simulink model "Flexible_Beam_Compare"  (R2016a)
settings: Solver=ode23t  StartTime=0.0  StopTime=10  MaxStep=5e-3  RelTol=1e-3  AbsTol=1e-3
PreLoadFcn:
  | Rigid_BoB = Simulink.Variant('Rigid_Body == 1');
  | Rigid_Link = Simulink.Variant('Rigid_Body == 2');
  | Rigid_Body = 1;
PostLoadFcn:
  | warning off Simulink:Engine:UsingDefaultMaxStepSize
  | warning off sm:compiler:topologyAnalysis:OnePortForceBlockGrounded
  | warning off Simulink:Parameters:ASTReadOnlyIfCompiledMaskField
  | warning off Simulink:Engine:SaveWithParameterizedLinks_Warning
  | warning off Simulink:Engine:OutputNotConnected
  | warning off Simulink:Engine:InputNotConnected
InitFcn:
  | %if ~exist('linsys_beam_fixfree','var') ||~exist('linsys_beam_rotfree','var')
  |    load SS_Damping_1e7.mat
  |    disp('State Space Models does not exist in workspace, loading presaved SS models')
  | %end
undefined symbols (not defined in the file or in its folder): beam_length, beam_wall, beam_width, density, element_length, Extr_Data_Box, gravity, Heavy_Weight, num_elem, X, Y, Z
undefined symbols (not defined in the file): Damping, kbendingx, kbendingy, kelongz, ktwistz, shearM, youngsM
libraries: sm_lib x240, nesl_utility x9, cstblocks x1
(part 1 of 7)
Description:
  | Copyright 2014-2016 The MathWorks, Inc.
settings Model: TunableVars=Heavy_Weight  TunableVarsStorageClass=Auto  Creator=smiller  LastModifiedBy=smiller
settings SolverCC: ZeroCrossAlgorithm=Adaptive
settings DataIOCC: LimitDataPoints=on  SaveFormat=Array
settings OptimizationCC: DefaultParameterBehavior=Inlined
settings DebuggingCC: AlgebraicLoopMsg=error  UnderspecifiedInitializationDetection=Classic  MergeDetectMultiDrivingBlocksExec=none  SolverPrmCheckMsg=warning  AllowSymbolicDim=off  StateNameClashWarn=warning
settings HardwareCC: ProdBitPerPointer=32  ProdLargestAtomicFloat=None  ProdIntDivRoundTo=Undefined  ProdEndianess=Unspecified  ProdWordSize=32  ProdHWDeviceType=32-bit Generic  TargetBitPerPointer=64  TargetLongLongMode=on  TargetIntDivRoundTo=Zero  TargetEndianess=LittleEndian  TargetWordSize=64  TargetHWDeviceType=MATLAB Host  ProdEqTarget=off
settings ModelReferenceCC: PropagateSignalLabelsOutOfModel=off
settings RTWCC: SystemTargetFile=rsim.tlc  TemplateMakefile=rsim_default_tmf  Description=Rapid Simulation Target
settings RSimTargetCC: ERTMultiwordTypeDef=System defined  ERTMultiwordLength=256
settings ConfigComp: CovModelRefEnable=Off  CovSFcnEnable=off
settings SimscapeCC: SimscapeLogLimitData=off
settings ConfigurationSet: Description=SimMechanics 2G
settings DiagnosticsConfigSet: SimMechanicsUnconnectedFramePorts=none  SimMechanicsRigidlyBoundBlock=warning
settings ExplorerConfigSet: InternalSimMechanicsExplorerSettings="<ExplorerConfiguration><canonicalview>default</canonicalview><AnimationSetting><BasePlaybackSpeed>1.0</BasePlaybackSpeed><PlaybackSpeedFactor>1.0</PlaybackSpeedFactor></AnimationSetting><TilePanel><TileInfo><Tiles Columns=\"1\" Count=\"1\" Rows=\"1\"><Column Left=\"2\" Weight=\"1\"/><Column Left=\"626\"/><Row Top=\"2\" Weight=\"1\"/><Row Top=\"393\"/><Tile Height=\"1\" Width=\"1\" X=\"0\" Y=\"0\"/></Tiles></TileInfo><SceneInfo><SceneViewer><BGColor><R>0.60000002384185791</R><G>0.60000002384185791</G><B>0.60000002384185791</B></BGColor><Camera><Position><X>49.330755486805451</X><Y>-0.55803913686158779</Y><Z>2.4998328760631781</Z></Position><Center><X>15.534556771714037</X><Y>-0.93059923918877141</Y><Z>0.031810436074220405</Z></Center><Up><X>-0.011334240993120652</X><Y>0.99992667770693056</Y><Z>0.004263119877513607</Z></Up><Left>-2.2154408151596012</Left><Right>2.2154408151596012</Right><Bottom>-1.878380911550241</Bottom><Top>1.878380911550241</Top></Camera></SceneViewer></SceneInfo></TilePanel></ExplorerConfiguration>"

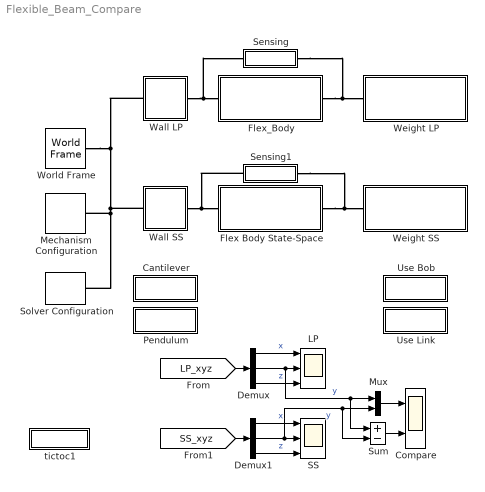
== system Flexible_Beam_Compare ==
  Cantilever : Subsystem
      settings: OpenFcn=|
      | set_param([bdroot '/Wall LP'],'OverrideUsingVariant','Fixed');
      | set_param([bdroot '/Wall SS'],'OverrideUsingVariant','Fixed');
      | 
      | LTIpth = find_system(bdroot,'ReferenceBlock','cstblocks/LTI System');
      | set_param(char(LTIpth),'sys','linsys_beam_fixfree');
      mask Display: disp('Cantilever');
  Compare : Scope  NumInputPorts=2
  Demux : Demux  Outputs=3
  Demux1 : Demux  Outputs=3
  Flex Body State-Space : Subsystem
      mask Display:
      | image(imread('SS_Beam.png'));
      | color red
      | port_label('LConn',1,'B');
      | port_label('RConn',1,'F');
  Flex_Body : Subsystem  mask(Flexible Body){rho=density, youngsM=youngsM, shearM=shearM, numelem=num_elem, beam_length=beam_length, beam_width=beam_width, beam_wall=beam_wall, b=Damping}
      mask prompts: rho "Material Density (kg/(m^3)"; youngsM "Modulus of Elasticity (N/m2)"; shearM "Shear Modulus (N/m2)"; numelem "Number of elements"; beam_length "Beam Length (m)"; beam_width "Beam Width & Height (m)"; beam_wall "Beam Wall Thickness(m)"; b "Damping Constant (Nm/rad.s)"
      mask help:
      | Models a flexible hollow square beam based on lumped parameter method.
      | Number of flexible elements, material properties as well as beam
      | dimension can be varied from mask parameters.
      mask init:
      | [kbendingx, kbendingy, ktwistz, kelongz, length] = Compute_GFE_Prop(rho, youngsM, shearM, numelem, beam_length, beam_width,beam_wall);
      | thisblock = gcb;
      | anno = ['No of Elem: ' num2str(numelem)];
      | set_param(thisblock, 'AttributesFormatString',anno);
      | if numelem <1
      |     error('Number of Flexible elements should be greater than 0')
      | end
      | prev_flex_bod = find_system(gcb,'LookUnderMasks','all','RegExp','on','Name','Flex_Elem_*');
      | if ~isempty(prev_flex_bod)
      |     delete_block(prev_flex_bod(1:end))
      | end
      | linehan = find_system(thisblock,'LookUnderMasks','all','FindAll','on','type','line');
      | if ~isempty(linehan)
      |     delete_line(linehan)
      | end
      | blk_or = [100 155 140 195];
      | set_param([thisblock '/B'],'Position',blk_or)
      | set_param([thisblock '/' sprintf('Transform\nBeamX')],'Position',blk_or+[80 0 80 0])
      | add_line(thisblock,['B/Rconn1'],[sprintf('Transform\nBeamX') '/Lconn1'],'autorouting','on');
      | add_block('FlexBeamElement_MS2G_Lib/Bend_Simple',[thisblock '/Flex_Elem_' num2str(1)],'Position',blk_or+[80 0 80 0]*2)
      | add_line(thisblock,[sprintf('Transform\nBeamX') '/Rconn1'],['Flex_Elem_' num2str(1) '/Lconn1'],'autorouting','on');
      | set_param([thisblock '/Flex_Elem_' num2str(1)], 'LinkStatus', 'none')
      | state_order{1} = [thisblock '/Flex_Elem_' num2str(1) '/Revolute Joint'];
      | for i = 2:1:numelem
      |     add_block('FlexBeamElement_MS2G_Lib/Bend_Simple',[thisblock '/Flex_Elem_' num2str(i)],'Position',blk_or+(i+1)*[80 0 80 0])
      |     add_line(thisblock,['Flex_Elem_' num2str(i-1) '/Rconn1'],['Flex_Elem_' num2str(i) '/Lconn1'],'autorouting','on');
      |     set_param([thisblock '/Flex_Elem_' num2str(i)], 'LinkStatus', 'none')
      |     state_order{i} = [thisblock '/Flex_Elem_' num2str(i) '/Revolute Joint'];
      | end
      | set_param([thisblock '/F'],'Position',blk_or+ (numelem+2)*[80 0 80 0]);
      | add_line(thisblock,['Flex_Elem_' num2str(numelem) '/Rconn1'],['F/Rconn1'],'autorouting','on');
      | assignin('base','State_order',state_order)
      settings: AttributesFormatString=No of Elem: 30  CopyFcn=set_param(gcb, 'LinkStatus', 'none')
      mask Display:
      | image(imread('Flexible_Beam.png'));
      | color red
      | port_label('LConn',1,'B');
      | port_label('RConn',1,'F');
  LP : Scope  NumInputPorts=3
  Mechanism Configuration : sm_lib/Utilities/Mechanism Configuration  UniformGravity=Constant  GravityVector=gravity  GravityUnits=m/s^2  LinearizationDelta=0.001
  Mux : Mux  Inputs=2
  Pendulum : Subsystem
      settings: OpenFcn=|
      | set_param([bdroot '/Wall LP'],'OverrideUsingVariant','Rotate');
      | set_param([bdroot '/Wall SS'],'OverrideUsingVariant','Rotate');
      | 
      | LTIpth = find_system(bdroot,'ReferenceBlock','cstblocks/LTI System');
      | set_param(char(LTIpth),'sys','linsys_beam_rotfree');
      mask Display: disp('Pendulum');
  SS : Scope  NumInputPorts=3
  Sensing : Subsystem
      mask Display: disp('S')
  Sensing1 : Subsystem
      mask Display: disp('S')
  Solver Configuration : nesl_utility/Solver Configuration  PhysicalDomain=network_engine_domain  SubClassName=solver  LeftPortType=input  RightPortType=generic  Accelerate=off  Tones=[]  Harmonics=[]  SimulateNoise=off  Profile=off  UseLocalSampling=off  EnableSwitchedLinearOptims=on  FrequencyDomain=off  UseCCode=off  RelTol=0.001  AbsTol=1e-06  MinStep=1e-09  ToWorkspace=off  RevertToSquareIcSolve=off  NumHomotopyIterations=100  PhasorMode=off  PhasorModeNumHarmonics=1  OverrideAbsTol=off  DoDC=off  ResidualTolerance=1e-09  UseLocalSolver=off  LocalSolverChoice=NE_BACKWARD_EULER_ADVANCER  LocalSolverSampleTime=0.001  DoFixedCost=off  MaxNonlinIter=3  MaxModeIter=2  LinearAlgebra=Sparse  DelaysMemoryBudget=1024  AutomaticFiltering=on  FilteringTimeConstant=0.001
  Sum : Sum  Inputs=+-
  Use Bob : Subsystem
      settings: OpenFcn=|
      | set_param([bdroot '/Weight LP'],'OverrideUsingVariant','Bob');
      | set_param([bdroot '/Weight SS'],'OverrideUsingVariant','Bob');
      mask Display: disp('Use Bob');
  Use Link : Subsystem
      settings: OpenFcn=|
      | set_param([bdroot '/Weight LP'],'OverrideUsingVariant','Link');
      | set_param([bdroot '/Weight SS'],'OverrideUsingVariant','Link');
      mask Display: disp('Use Link');
  Wall LP : Subsystem  Variant=on  OverrideUsingVariant=Fixed
      mask Display:
      | if strcmp(get_param(gcb,'ActiveVariant'),'Fixed')
      |     image(imread('Weld_Image.png'))
      | else
      |     image(imread('Rev_Image.png'))
      | end
      | color red
      | port_label('LConn',1,'B');
      | port_label('Rconn',1,'F');
  Wall SS : Subsystem  Variant=on  OverrideUsingVariant=Fixed
      mask Display:
      | if strcmp(get_param(gcb,'ActiveVariant'),'Fixed')
      |     image(imread('Weld_Image.png'))
      | else
      |     image(imread('Rev_Image.png'))
      | end
      | color red
      | port_label('LConn',1,'B');
      | port_label('Rconn',1,'F');
  Weight LP : Subsystem  Variant=on  OverrideUsingVariant=Bob
      mask Display:
      | if strcmp(get_param(gcb,'ActiveVariant'),'Bob')
      |     image(imread('BOB_LP.png'))
      | else
      |     image(imread('Link.png'))
      | end
      | color red
      | port_label('LConn',1,'B');
      | port_label('Rconn',1,'F');
  Weight SS : Subsystem  Variant=on  OverrideUsingVariant=Bob
      mask Display:
      | if strcmp(get_param(gcb,'ActiveVariant'),'Bob')
      |     image(imread('BOB.png'))
      | else
      |     image(imread('Link.png'))
      | end
      | color red
      | port_label('LConn',1,'B');
      | port_label('Rconn',1,'F');
  World Frame : sm_lib/Frames and Transforms/World Frame
  tictoc1 : Subsystem
      settings: OpenFcn=open('Flexible_Beam_Demo_Script.html')
      mask Display: disp('Script')
  wires:
  Demux/1 -> LP/1  "x"
  Demux/2 -> Sum/1, Mux/1, LP/2  "y"
  Demux/3 -> LP/3  "z"
  Demux1/1 -> SS/1  "x"
  Demux1/2 -> SS/2, Sum/2, Mux/2  "y"
  Demux1/3 -> SS/3  "z"
  Mux/1 -> Compare/1
  Sum/1 -> Compare/2
  [LP_xyz] -> Demux/1
  [SS_xyz] -> Demux1/1
  connections:
  Solver Configuration/RConn1 -- Wall LP/LConn1 -- World Frame/RConn1 -- Wall SS/LConn1 -- Mechanism Configuration/RConn1
  Sensing/LConn1 -- Flex_Body/RConn1 -- Weight LP/LConn1
  Flex Body State-Space/RConn1 -- Sensing1/LConn1 -- Weight SS/LConn1
  Wall LP/RConn1 -- Flex_Body/LConn1 -- Sensing/RConn1
  Wall SS/RConn1 -- Sensing1/RConn1 -- Flex Body State-Space/LConn1

== system Flexible_Beam_Compare/Cantilever ==

== system Flexible_Beam_Compare/Flex Body State-Space ==
  Deflection Joint : Subsystem
  Rigid Body : Subsystem
  State-Space Model : Subsystem
  B : PMIOPort  Port=1  Side=Left
  F : PMIOPort  Port=2  Side=Right
  connections:
  Deflection Joint/RConn2 -- F/RConn1
  Rigid Body/LConn1 -- B/RConn1
  Deflection Joint/LConn2 -- Rigid Body/RConn1
  State-Space Model/RConn1 -- Deflection Joint/LConn1
  State-Space Model/LConn1 -- Deflection Joint/RConn1

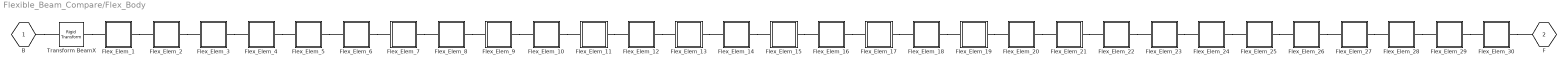
== system Flexible_Beam_Compare/Flex_Body ==
  Flex_Elem_1 : Subsystem  mask{length=length, rho=rho, beam_width=beam_width, beam_wall=beam_wall, kbendingx=kbendingx, kbendingy=kbendingy, kbendingz=ktwistz, kelongz=kelongz, b=b}
      mask prompts: length "Beam Length (m)"; rho "Material Density (kg/(m^3)"; beam_width "Beam Width & Height (m)"; beam_wall "Beam Wall Thickness (m)"; kbendingx "Bending Spring Constant about X(Nm/rad)"; kbendingy "Bending Spring Constant about Y(Nm/rad)"; kbendingz "Twist Spring Constant about Z(Nm/rad)"; kelongz "Elongation Spring Constant about Z(N/m)"; b "Damping Constant (Nm/rad.s)"
  Flex_Elem_10 : Subsystem  mask{length=length, rho=rho, beam_width=beam_width, beam_wall=beam_wall, kbendingx=kbendingx, kbendingy=kbendingy, kbendingz=ktwistz, kelongz=kelongz, b=b}
      mask prompts: length "Beam Length (m)"; rho "Material Density (kg/(m^3)"; beam_width "Beam Width & Height (m)"; beam_wall "Beam Wall Thickness (m)"; kbendingx "Bending Spring Constant about X(Nm/rad)"; kbendingy "Bending Spring Constant about Y(Nm/rad)"; kbendingz "Twist Spring Constant about Z(Nm/rad)"; kelongz "Elongation Spring Constant about Z(N/m)"; b "Damping Constant (Nm/rad.s)"
  Flex_Elem_11 : Subsystem  mask{length=length, rho=rho, beam_width=beam_width, beam_wall=beam_wall, kbendingx=kbendingx, kbendingy=kbendingy, kbendingz=ktwistz, kelongz=kelongz, b=b}
      mask prompts: length "Beam Length (m)"; rho "Material Density (kg/(m^3)"; beam_width "Beam Width & Height (m)"; beam_wall "Beam Wall Thickness (m)"; kbendingx "Bending Spring Constant about X(Nm/rad)"; kbendingy "Bending Spring Constant about Y(Nm/rad)"; kbendingz "Twist Spring Constant about Z(Nm/rad)"; kelongz "Elongation Spring Constant about Z(N/m)"; b "Damping Constant (Nm/rad.s)"
  Flex_Elem_12 : Subsystem  mask{length=length, rho=rho, beam_width=beam_width, beam_wall=beam_wall, kbendingx=kbendingx, kbendingy=kbendingy, kbendingz=ktwistz, kelongz=kelongz, b=b}
      mask prompts: length "Beam Length (m)"; rho "Material Density (kg/(m^3)"; beam_width "Beam Width & Height (m)"; beam_wall "Beam Wall Thickness (m)"; kbendingx "Bending Spring Constant about X(Nm/rad)"; kbendingy "Bending Spring Constant about Y(Nm/rad)"; kbendingz "Twist Spring Constant about Z(Nm/rad)"; kelongz "Elongation Spring Constant about Z(N/m)"; b "Damping Constant (Nm/rad.s)"
  Flex_Elem_13 : Subsystem  mask{length=length, rho=rho, beam_width=beam_width, beam_wall=beam_wall, kbendingx=kbendingx, kbendingy=kbendingy, kbendingz=ktwistz, kelongz=kelongz, b=b}
      mask prompts: length "Beam Length (m)"; rho "Material Density (kg/(m^3)"; beam_width "Beam Width & Height (m)"; beam_wall "Beam Wall Thickness (m)"; kbendingx "Bending Spring Constant about X(Nm/rad)"; kbendingy "Bending Spring Constant about Y(Nm/rad)"; kbendingz "Twist Spring Constant about Z(Nm/rad)"; kelongz "Elongation Spring Constant about Z(N/m)"; b "Damping Constant (Nm/rad.s)"
  Flex_Elem_14 : Subsystem  mask{length=length, rho=rho, beam_width=beam_width, beam_wall=beam_wall, kbendingx=kbendingx, kbendingy=kbendingy, kbendingz=ktwistz, kelongz=kelongz, b=b}
      mask prompts: length "Beam Length (m)"; rho "Material Density (kg/(m^3)"; beam_width "Beam Width & Height (m)"; beam_wall "Beam Wall Thickness (m)"; kbendingx "Bending Spring Constant about X(Nm/rad)"; kbendingy "Bending Spring Constant about Y(Nm/rad)"; kbendingz "Twist Spring Constant about Z(Nm/rad)"; kelongz "Elongation Spring Constant about Z(N/m)"; b "Damping Constant (Nm/rad.s)"
  Flex_Elem_15 : Subsystem  mask{length=length, rho=rho, beam_width=beam_width, beam_wall=beam_wall, kbendingx=kbendingx, kbendingy=kbendingy, kbendingz=ktwistz, kelongz=kelongz, b=b}
      mask prompts: length "Beam Length (m)"; rho "Material Density (kg/(m^3)"; beam_width "Beam Width & Height (m)"; beam_wall "Beam Wall Thickness (m)"; kbendingx "Bending Spring Constant about X(Nm/rad)"; kbendingy "Bending Spring Constant about Y(Nm/rad)"; kbendingz "Twist Spring Constant about Z(Nm/rad)"; kelongz "Elongation Spring Constant about Z(N/m)"; b "Damping Constant (Nm/rad.s)"
  Flex_Elem_16 : Subsystem  mask{length=length, rho=rho, beam_width=beam_width, beam_wall=beam_wall, kbendingx=kbendingx, kbendingy=kbendingy, kbendingz=ktwistz, kelongz=kelongz, b=b}
      mask prompts: length "Beam Length (m)"; rho "Material Density (kg/(m^3)"; beam_width "Beam Width & Height (m)"; beam_wall "Beam Wall Thickness (m)"; kbendingx "Bending Spring Constant about X(Nm/rad)"; kbendingy "Bending Spring Constant about Y(Nm/rad)"; kbendingz "Twist Spring Constant about Z(Nm/rad)"; kelongz "Elongation Spring Constant about Z(N/m)"; b "Damping Constant (Nm/rad.s)"
  Flex_Elem_17 : Subsystem  mask{length=length, rho=rho, beam_width=beam_width, beam_wall=beam_wall, kbendingx=kbendingx, kbendingy=kbendingy, kbendingz=ktwistz, kelongz=kelongz, b=b}
      mask prompts: length "Beam Length (m)"; rho "Material Density (kg/(m^3)"; beam_width "Beam Width & Height (m)"; beam_wall "Beam Wall Thickness (m)"; kbendingx "Bending Spring Constant about X(Nm/rad)"; kbendingy "Bending Spring Constant about Y(Nm/rad)"; kbendingz "Twist Spring Constant about Z(Nm/rad)"; kelongz "Elongation Spring Constant about Z(N/m)"; b "Damping Constant (Nm/rad.s)"
  Flex_Elem_18 : Subsystem  mask{length=length, rho=rho, beam_width=beam_width, beam_wall=beam_wall, kbendingx=kbendingx, kbendingy=kbendingy, kbendingz=ktwistz, kelongz=kelongz, b=b}
      mask prompts: length "Beam Length (m)"; rho "Material Density (kg/(m^3)"; beam_width "Beam Width & Height (m)"; beam_wall "Beam Wall Thickness (m)"; kbendingx "Bending Spring Constant about X(Nm/rad)"; kbendingy "Bending Spring Constant about Y(Nm/rad)"; kbendingz "Twist Spring Constant about Z(Nm/rad)"; kelongz "Elongation Spring Constant about Z(N/m)"; b "Damping Constant (Nm/rad.s)"
  Flex_Elem_19 : Subsystem  mask{length=length, rho=rho, beam_width=beam_width, beam_wall=beam_wall, kbendingx=kbendingx, kbendingy=kbendingy, kbendingz=ktwistz, kelongz=kelongz, b=b}
      mask prompts: length "Beam Length (m)"; rho "Material Density (kg/(m^3)"; beam_width "Beam Width & Height (m)"; beam_wall "Beam Wall Thickness (m)"; kbendingx "Bending Spring Constant about X(Nm/rad)"; kbendingy "Bending Spring Constant about Y(Nm/rad)"; kbendingz "Twist Spring Constant about Z(Nm/rad)"; kelongz "Elongation Spring Constant about Z(N/m)"; b "Damping Constant (Nm/rad.s)"
  Flex_Elem_2 : Subsystem  mask{length=length, rho=rho, beam_width=beam_width, beam_wall=beam_wall, kbendingx=kbendingx, kbendingy=kbendingy, kbendingz=ktwistz, kelongz=kelongz, b=b}
      mask prompts: length "Beam Length (m)"; rho "Material Density (kg/(m^3)"; beam_width "Beam Width & Height (m)"; beam_wall "Beam Wall Thickness (m)"; kbendingx "Bending Spring Constant about X(Nm/rad)"; kbendingy "Bending Spring Constant about Y(Nm/rad)"; kbendingz "Twist Spring Constant about Z(Nm/rad)"; kelongz "Elongation Spring Constant about Z(N/m)"; b "Damping Constant (Nm/rad.s)"
  Flex_Elem_20 : Subsystem  mask{length=length, rho=rho, beam_width=beam_width, beam_wall=beam_wall, kbendingx=kbendingx, kbendingy=kbendingy, kbendingz=ktwistz, kelongz=kelongz, b=b}
      mask prompts: length "Beam Length (m)"; rho "Material Density (kg/(m^3)"; beam_width "Beam Width & Height (m)"; beam_wall "Beam Wall Thickness (m)"; kbendingx "Bending Spring Constant about X(Nm/rad)"; kbendingy "Bending Spring Constant about Y(Nm/rad)"; kbendingz "Twist Spring Constant about Z(Nm/rad)"; kelongz "Elongation Spring Constant about Z(N/m)"; b "Damping Constant (Nm/rad.s)"
  Flex_Elem_21 : Subsystem  mask{length=length, rho=rho, beam_width=beam_width, beam_wall=beam_wall, kbendingx=kbendingx, kbendingy=kbendingy, kbendingz=ktwistz, kelongz=kelongz, b=b}
      mask prompts: length "Beam Length (m)"; rho "Material Density (kg/(m^3)"; beam_width "Beam Width & Height (m)"; beam_wall "Beam Wall Thickness (m)"; kbendingx "Bending Spring Constant about X(Nm/rad)"; kbendingy "Bending Spring Constant about Y(Nm/rad)"; kbendingz "Twist Spring Constant about Z(Nm/rad)"; kelongz "Elongation Spring Constant about Z(N/m)"; b "Damping Constant (Nm/rad.s)"
  Flex_Elem_22 : Subsystem  mask{length=length, rho=rho, beam_width=beam_width, beam_wall=beam_wall, kbendingx=kbendingx, kbendingy=kbendingy, kbendingz=ktwistz, kelongz=kelongz, b=b}
      mask prompts: length "Beam Length (m)"; rho "Material Density (kg/(m^3)"; beam_width "Beam Width & Height (m)"; beam_wall "Beam Wall Thickness (m)"; kbendingx "Bending Spring Constant about X(Nm/rad)"; kbendingy "Bending Spring Constant about Y(Nm/rad)"; kbendingz "Twist Spring Constant about Z(Nm/rad)"; kelongz "Elongation Spring Constant about Z(N/m)"; b "Damping Constant (Nm/rad.s)"
  Flex_Elem_23 : Subsystem  mask{length=length, rho=rho, beam_width=beam_width, beam_wall=beam_wall, kbendingx=kbendingx, kbendingy=kbendingy, kbendingz=ktwistz, kelongz=kelongz, b=b}
      mask prompts: length "Beam Length (m)"; rho "Material Density (kg/(m^3)"; beam_width "Beam Width & Height (m)"; beam_wall "Beam Wall Thickness (m)"; kbendingx "Bending Spring Constant about X(Nm/rad)"; kbendingy "Bending Spring Constant about Y(Nm/rad)"; kbendingz "Twist Spring Constant about Z(Nm/rad)"; kelongz "Elongation Spring Constant about Z(N/m)"; b "Damping Constant (Nm/rad.s)"
  Flex_Elem_24 : Subsystem  mask{length=length, rho=rho, beam_width=beam_width, beam_wall=beam_wall, kbendingx=kbendingx, kbendingy=kbendingy, kbendingz=ktwistz, kelongz=kelongz, b=b}
      mask prompts: length "Beam Length (m)"; rho "Material Density (kg/(m^3)"; beam_width "Beam Width & Height (m)"; beam_wall "Beam Wall Thickness (m)"; kbendingx "Bending Spring Constant about X(Nm/rad)"; kbendingy "Bending Spring Constant about Y(Nm/rad)"; kbendingz "Twist Spring Constant about Z(Nm/rad)"; kelongz "Elongation Spring Constant about Z(N/m)"; b "Damping Constant (Nm/rad.s)"
  Flex_Elem_25 : Subsystem  mask{length=length, rho=rho, beam_width=beam_width, beam_wall=beam_wall, kbendingx=kbendingx, kbendingy=kbendingy, kbendingz=ktwistz, kelongz=kelongz, b=b}
      mask prompts: length "Beam Length (m)"; rho "Material Density (kg/(m^3)"; beam_width "Beam Width & Height (m)"; beam_wall "Beam Wall Thickness (m)"; kbendingx "Bending Spring Constant about X(Nm/rad)"; kbendingy "Bending Spring Constant about Y(Nm/rad)"; kbendingz "Twist Spring Constant about Z(Nm/rad)"; kelongz "Elongation Spring Constant about Z(N/m)"; b "Damping Constant (Nm/rad.s)"
  Flex_Elem_26 : Subsystem  mask{length=length, rho=rho, beam_width=beam_width, beam_wall=beam_wall, kbendingx=kbendingx, kbendingy=kbendingy, kbendingz=ktwistz, kelongz=kelongz, b=b}
      mask prompts: length "Beam Length (m)"; rho "Material Density (kg/(m^3)"; beam_width "Beam Width & Height (m)"; beam_wall "Beam Wall Thickness (m)"; kbendingx "Bending Spring Constant about X(Nm/rad)"; kbendingy "Bending Spring Constant about Y(Nm/rad)"; kbendingz "Twist Spring Constant about Z(Nm/rad)"; kelongz "Elongation Spring Constant about Z(N/m)"; b "Damping Constant (Nm/rad.s)"
  Flex_Elem_27 : Subsystem  mask{length=length, rho=rho, beam_width=beam_width, beam_wall=beam_wall, kbendingx=kbendingx, kbendingy=kbendingy, kbendingz=ktwistz, kelongz=kelongz, b=b}
      mask prompts: length "Beam Length (m)"; rho "Material Density (kg/(m^3)"; beam_width "Beam Width & Height (m)"; beam_wall "Beam Wall Thickness (m)"; kbendingx "Bending Spring Constant about X(Nm/rad)"; kbendingy "Bending Spring Constant about Y(Nm/rad)"; kbendingz "Twist Spring Constant about Z(Nm/rad)"; kelongz "Elongation Spring Constant about Z(N/m)"; b "Damping Constant (Nm/rad.s)"
  Flex_Elem_28 : Subsystem  mask{length=length, rho=rho, beam_width=beam_width, beam_wall=beam_wall, kbendingx=kbendingx, kbendingy=kbendingy, kbendingz=ktwistz, kelongz=kelongz, b=b}
      mask prompts: length "Beam Length (m)"; rho "Material Density (kg/(m^3)"; beam_width "Beam Width & Height (m)"; beam_wall "Beam Wall Thickness (m)"; kbendingx "Bending Spring Constant about X(Nm/rad)"; kbendingy "Bending Spring Constant about Y(Nm/rad)"; kbendingz "Twist Spring Constant about Z(Nm/rad)"; kelongz "Elongation Spring Constant about Z(N/m)"; b "Damping Constant (Nm/rad.s)"
  Flex_Elem_29 : Subsystem  mask{length=length, rho=rho, beam_width=beam_width, beam_wall=beam_wall, kbendingx=kbendingx, kbendingy=kbendingy, kbendingz=ktwistz, kelongz=kelongz, b=b}
      mask prompts: length "Beam Length (m)"; rho "Material Density (kg/(m^3)"; beam_width "Beam Width & Height (m)"; beam_wall "Beam Wall Thickness (m)"; kbendingx "Bending Spring Constant about X(Nm/rad)"; kbendingy "Bending Spring Constant about Y(Nm/rad)"; kbendingz "Twist Spring Constant about Z(Nm/rad)"; kelongz "Elongation Spring Constant about Z(N/m)"; b "Damping Constant (Nm/rad.s)"
  Flex_Elem_3 : Subsystem  mask{length=length, rho=rho, beam_width=beam_width, beam_wall=beam_wall, kbendingx=kbendingx, kbendingy=kbendingy, kbendingz=ktwistz, kelongz=kelongz, b=b}
      mask prompts: length "Beam Length (m)"; rho "Material Density (kg/(m^3)"; beam_width "Beam Width & Height (m)"; beam_wall "Beam Wall Thickness (m)"; kbendingx "Bending Spring Constant about X(Nm/rad)"; kbendingy "Bending Spring Constant about Y(Nm/rad)"; kbendingz "Twist Spring Constant about Z(Nm/rad)"; kelongz "Elongation Spring Constant about Z(N/m)"; b "Damping Constant (Nm/rad.s)"
  Flex_Elem_30 : Subsystem  mask{length=length, rho=rho, beam_width=beam_width, beam_wall=beam_wall, kbendingx=kbendingx, kbendingy=kbendingy, kbendingz=ktwistz, kelongz=kelongz, b=b}
      mask prompts: length "Beam Length (m)"; rho "Material Density (kg/(m^3)"; beam_width "Beam Width & Height (m)"; beam_wall "Beam Wall Thickness (m)"; kbendingx "Bending Spring Constant about X(Nm/rad)"; kbendingy "Bending Spring Constant about Y(Nm/rad)"; kbendingz "Twist Spring Constant about Z(Nm/rad)"; kelongz "Elongation Spring Constant about Z(N/m)"; b "Damping Constant (Nm/rad.s)"
  Flex_Elem_4 : Subsystem  mask{length=length, rho=rho, beam_width=beam_width, beam_wall=beam_wall, kbendingx=kbendingx, kbendingy=kbendingy, kbendingz=ktwistz, kelongz=kelongz, b=b}
      mask prompts: length "Beam Length (m)"; rho "Material Density (kg/(m^3)"; beam_width "Beam Width & Height (m)"; beam_wall "Beam Wall Thickness (m)"; kbendingx "Bending Spring Constant about X(Nm/rad)"; kbendingy "Bending Spring Constant about Y(Nm/rad)"; kbendingz "Twist Spring Constant about Z(Nm/rad)"; kelongz "Elongation Spring Constant about Z(N/m)"; b "Damping Constant (Nm/rad.s)"
  Flex_Elem_5 : Subsystem  mask{length=length, rho=rho, beam_width=beam_width, beam_wall=beam_wall, kbendingx=kbendingx, kbendingy=kbendingy, kbendingz=ktwistz, kelongz=kelongz, b=b}
      mask prompts: length "Beam Length (m)"; rho "Material Density (kg/(m^3)"; beam_width "Beam Width & Height (m)"; beam_wall "Beam Wall Thickness (m)"; kbendingx "Bending Spring Constant about X(Nm/rad)"; kbendingy "Bending Spring Constant about Y(Nm/rad)"; kbendingz "Twist Spring Constant about Z(Nm/rad)"; kelongz "Elongation Spring Constant about Z(N/m)"; b "Damping Constant (Nm/rad.s)"
  Flex_Elem_6 : Subsystem  mask{length=length, rho=rho, beam_width=beam_width, beam_wall=beam_wall, kbendingx=kbendingx, kbendingy=kbendingy, kbendingz=ktwistz, kelongz=kelongz, b=b}
      mask prompts: length "Beam Length (m)"; rho "Material Density (kg/(m^3)"; beam_width "Beam Width & Height (m)"; beam_wall "Beam Wall Thickness (m)"; kbendingx "Bending Spring Constant about X(Nm/rad)"; kbendingy "Bending Spring Constant about Y(Nm/rad)"; kbendingz "Twist Spring Constant about Z(Nm/rad)"; kelongz "Elongation Spring Constant about Z(N/m)"; b "Damping Constant (Nm/rad.s)"
  Flex_Elem_7 : Subsystem  mask{length=length, rho=rho, beam_width=beam_width, beam_wall=beam_wall, kbendingx=kbendingx, kbendingy=kbendingy, kbendingz=ktwistz, kelongz=kelongz, b=b}
      mask prompts: length "Beam Length (m)"; rho "Material Density (kg/(m^3)"; beam_width "Beam Width & Height (m)"; beam_wall "Beam Wall Thickness (m)"; kbendingx "Bending Spring Constant about X(Nm/rad)"; kbendingy "Bending Spring Constant about Y(Nm/rad)"; kbendingz "Twist Spring Constant about Z(Nm/rad)"; kelongz "Elongation Spring Constant about Z(N/m)"; b "Damping Constant (Nm/rad.s)"
  Flex_Elem_8 : Subsystem  mask{length=length, rho=rho, beam_width=beam_width, beam_wall=beam_wall, kbendingx=kbendingx, kbendingy=kbendingy, kbendingz=ktwistz, kelongz=kelongz, b=b}
      mask prompts: length "Beam Length (m)"; rho "Material Density (kg/(m^3)"; beam_width "Beam Width & Height (m)"; beam_wall "Beam Wall Thickness (m)"; kbendingx "Bending Spring Constant about X(Nm/rad)"; kbendingy "Bending Spring Constant about Y(Nm/rad)"; kbendingz "Twist Spring Constant about Z(Nm/rad)"; kelongz "Elongation Spring Constant about Z(N/m)"; b "Damping Constant (Nm/rad.s)"
  Flex_Elem_9 : Subsystem  mask{length=length, rho=rho, beam_width=beam_width, beam_wall=beam_wall, kbendingx=kbendingx, kbendingy=kbendingy, kbendingz=ktwistz, kelongz=kelongz, b=b}
      mask prompts: length "Beam Length (m)"; rho "Material Density (kg/(m^3)"; beam_width "Beam Width & Height (m)"; beam_wall "Beam Wall Thickness (m)"; kbendingx "Bending Spring Constant about X(Nm/rad)"; kbendingy "Bending Spring Constant about Y(Nm/rad)"; kbendingz "Twist Spring Constant about Z(Nm/rad)"; kelongz "Elongation Spring Constant about Z(N/m)"; b "Damping Constant (Nm/rad.s)"
  Transform BeamX : sm_lib/Frames and Transforms/Rigid Transform  TranslationMethod=StandardAxis  TranslationLengthUnit=m  TranslationStandardAxis=+Z  TranslationStandardOffset=0  TranslationCartesianOffset=[0 0 0]  TranslationROffset=0  TranslationROffsetUnits=m  TranslationZOffset=0  TranslationZOffsetUnits=m  TranslationThetaOffset=0  TranslationThetaOffsetUnits=deg  RotationMethod=StandardAxis  RotationAngleUnits=deg  RotationStandardAxis=+Y  RotationAngle=90  RotationArbitraryAxis=[0 0 1]  FollAlignAxisA=+X  BaseAlignAxisA=+Y  FollAlignAxisB=+Y  BaseAlignAxisB=+Z  RotationSequenceAxes=FollowerAxes  RotationSequence=XYX  RotationSequenceAngles=[0 0 0]  RotationSequenceAnglesUnits=deg  RotationMatrix=[1 0 0; 0 1 0; 0 0 1]
  B : PMIOPort  Port=1  Side=Left
  F : PMIOPort  Port=2  Side=Right
  connections:
  B/RConn1 -- Transform BeamX/LConn1
  Transform BeamX/RConn1 -- Flex_Elem_1/LConn1
  Flex_Elem_1/RConn1 -- Flex_Elem_2/LConn1
  Flex_Elem_2/RConn1 -- Flex_Elem_3/LConn1
  Flex_Elem_3/RConn1 -- Flex_Elem_4/LConn1
  Flex_Elem_4/RConn1 -- Flex_Elem_5/LConn1
  Flex_Elem_5/RConn1 -- Flex_Elem_6/LConn1
  Flex_Elem_6/RConn1 -- Flex_Elem_7/LConn1
  Flex_Elem_7/RConn1 -- Flex_Elem_8/LConn1
  Flex_Elem_8/RConn1 -- Flex_Elem_9/LConn1
  Flex_Elem_9/RConn1 -- Flex_Elem_10/LConn1
  Flex_Elem_10/RConn1 -- Flex_Elem_11/LConn1
  Flex_Elem_11/RConn1 -- Flex_Elem_12/LConn1
  Flex_Elem_12/RConn1 -- Flex_Elem_13/LConn1
  Flex_Elem_13/RConn1 -- Flex_Elem_14/LConn1
  Flex_Elem_14/RConn1 -- Flex_Elem_15/LConn1
  Flex_Elem_15/RConn1 -- Flex_Elem_16/LConn1
  Flex_Elem_16/RConn1 -- Flex_Elem_17/LConn1
  Flex_Elem_17/RConn1 -- Flex_Elem_18/LConn1
  Flex_Elem_18/RConn1 -- Flex_Elem_19/LConn1
  Flex_Elem_19/RConn1 -- Flex_Elem_20/LConn1
  Flex_Elem_20/RConn1 -- Flex_Elem_21/LConn1
  Flex_Elem_21/RConn1 -- Flex_Elem_22/LConn1
  Flex_Elem_22/RConn1 -- Flex_Elem_23/LConn1
  Flex_Elem_23/RConn1 -- Flex_Elem_24/LConn1
  Flex_Elem_24/RConn1 -- Flex_Elem_25/LConn1
  Flex_Elem_25/RConn1 -- Flex_Elem_26/LConn1
  Flex_Elem_26/RConn1 -- Flex_Elem_27/LConn1
  Flex_Elem_27/RConn1 -- Flex_Elem_28/LConn1
  Flex_Elem_28/RConn1 -- Flex_Elem_29/LConn1
  Flex_Elem_29/RConn1 -- Flex_Elem_30/LConn1
  Flex_Elem_30/RConn1 -- F/RConn1

== system Flexible_Beam_Compare/Pendulum ==

== system Flexible_Beam_Compare/Sensing ==
  Mux : Mux  Inputs=3
  PS-Simulink Converter : nesl_utility/PS-Simulink Converter  PhysicalDomain=network_engine_domain  SubClassName=ps_output  LeftPortType=input  RightPortType=output  PseudoPeriodic=off  Frequencies=[]  Unit=1  AffineConversion=off
  PS-Simulink Converter1 : nesl_utility/PS-Simulink Converter  PhysicalDomain=network_engine_domain  SubClassName=ps_output  LeftPortType=input  RightPortType=output  PseudoPeriodic=off  Frequencies=[]  Unit=1  AffineConversion=off
  PS-Simulink Converter2 : nesl_utility/PS-Simulink Converter  PhysicalDomain=network_engine_domain  SubClassName=ps_output  LeftPortType=input  RightPortType=output  PseudoPeriodic=off  Frequencies=[]  Unit=1  AffineConversion=off
  Transform Sensor : sm_lib/Frames and Transforms/Transform Sensor  MeasurementFrame=Base  SenseAngle=off  SenseAxis=off  SenseAngle1=off  SenseAngle2=off  SenseAngle3=off  SenseQ=off  SenseR=off  SenseOmegaX=off  SenseOmegaY=off  SenseOmegaZ=off  SenseOmega1=off  SenseOmega2=off  SenseOmega3=off  SenseQDot=off  SenseRDot=off  SenseAlphaX=off  SenseAlphaY=off  SenseAlphaZ=off  SenseAlpha1=off  SenseAlpha2=off  SenseAlpha3=off  SenseQDDot=off  SenseRDDot=off  SenseX=on  SenseY=on  SenseZ=on  SenseRad=off  SenseAzim=off  SenseDist=off  SenseInc=off  SenseXDot=off  SenseYDot=off  SenseZDot=off  SenseRadDot=off  SenseAzimDot=off  SenseDistDot=off  SenseIncDot=off  SenseXDDot=off  SenseYDDot=off  SenseZDDot=off  SenseRadDDot=off  SenseAzimDDot=off  SenseDistDDot=off  SenseIncDDot=off
  F : PMIOPort  Port=1  Side=Left
  B : PMIOPort  Port=2  Side=Right
  tag scope: LP_xyz=global
  wires:
  PS-Simulink Converter1/1 -> Mux/2
  PS-Simulink Converter2/1 -> Mux/3
  PS-Simulink Converter/1 -> Mux/1
  Mux/1 -> [LP_xyz]
  connections:
  PS-Simulink Converter2/LConn1 -- Transform Sensor/RConn4
  PS-Simulink Converter/LConn1 -- Transform Sensor/RConn2
  PS-Simulink Converter1/LConn1 -- Transform Sensor/RConn3
  B/RConn1 -- Transform Sensor/LConn1
  F/RConn1 -- Transform Sensor/RConn1

== system Flexible_Beam_Compare/Sensing1 ==
  Mux : Mux  Inputs=3
  PS-Simulink Converter : nesl_utility/PS-Simulink Converter  PhysicalDomain=network_engine_domain  SubClassName=ps_output  LeftPortType=input  RightPortType=output  PseudoPeriodic=off  Frequencies=[]  Unit=1  AffineConversion=off
  PS-Simulink Converter1 : nesl_utility/PS-Simulink Converter  PhysicalDomain=network_engine_domain  SubClassName=ps_output  LeftPortType=input  RightPortType=output  PseudoPeriodic=off  Frequencies=[]  Unit=1  AffineConversion=off
  PS-Simulink Converter2 : nesl_utility/PS-Simulink Converter  PhysicalDomain=network_engine_domain  SubClassName=ps_output  LeftPortType=input  RightPortType=output  PseudoPeriodic=off  Frequencies=[]  Unit=1  AffineConversion=off
  Transform Sensor : sm_lib/Frames and Transforms/Transform Sensor  MeasurementFrame=Base  SenseAngle=off  SenseAxis=off  SenseAngle1=off  SenseAngle2=off  SenseAngle3=off  SenseQ=off  SenseR=off  SenseOmegaX=off  SenseOmegaY=off  SenseOmegaZ=off  SenseOmega1=off  SenseOmega2=off  SenseOmega3=off  SenseQDot=off  SenseRDot=off  SenseAlphaX=off  SenseAlphaY=off  SenseAlphaZ=off  SenseAlpha1=off  SenseAlpha2=off  SenseAlpha3=off  SenseQDDot=off  SenseRDDot=off  SenseX=on  SenseY=on  SenseZ=on  SenseRad=off  SenseAzim=off  SenseDist=off  SenseInc=off  SenseXDot=off  SenseYDot=off  SenseZDot=off  SenseRadDot=off  SenseAzimDot=off  SenseDistDot=off  SenseIncDot=off  SenseXDDot=off  SenseYDDot=off  SenseZDDot=off  SenseRadDDot=off  SenseAzimDDot=off  SenseDistDDot=off  SenseIncDDot=off
  F : PMIOPort  Port=1  Side=Left
  B : PMIOPort  Port=2  Side=Right
  tag scope: SS_xyz=global
  wires:
  Mux/1 -> [SS_xyz]
  PS-Simulink Converter/1 -> Mux/1
  PS-Simulink Converter2/1 -> Mux/3
  PS-Simulink Converter1/1 -> Mux/2
  connections:
  F/RConn1 -- Transform Sensor/RConn1
  B/RConn1 -- Transform Sensor/LConn1
  PS-Simulink Converter1/LConn1 -- Transform Sensor/RConn3
  PS-Simulink Converter/LConn1 -- Transform Sensor/RConn2
  PS-Simulink Converter2/LConn1 -- Transform Sensor/RConn4

== system Flexible_Beam_Compare/Use Bob ==

== system Flexible_Beam_Compare/Use Link ==

== system Flexible_Beam_Compare/Wall LP ==
  note: 1) Only subsystems can be added as variant choices at this level
      | 2) Blocks cannot be connected at this level as connectivity is
      | automatically determined at simulation, based on the active variant
  Fixed : Subsystem  VariantControl=Fixed
  Rotate : Subsystem  VariantControl=Rotate
  B : PMIOPort  Port=1  Side=Left
  F : PMIOPort  Port=2  Side=Right

== system Flexible_Beam_Compare/Wall SS ==
  note: 1) Only subsystems can be added as variant choices at this level
      | 2) Blocks cannot be connected at this level as connectivity is
      | automatically determined at simulation, based on the active variant
  Fixed : Subsystem  VariantControl=Fixed
  Rotate : Subsystem  VariantControl=Rotate
  B : PMIOPort  Port=1  Side=Left
  F : PMIOPort  Port=2  Side=Right

== system Flexible_Beam_Compare/Weight LP ==
  note: 1) Only subsystems can be added as variant choices at this level
      | 2) Blocks cannot be connected at this level as connectivity is
      | automatically determined at simulation, based on the active variant
  Bob : Subsystem  VariantControl=Bob
  Link : Subsystem  VariantControl=Link
  B : PMIOPort  Port=1  Side=Left
  F : PMIOPort  Port=2  Side=Right

== system Flexible_Beam_Compare/Weight SS ==
  note: 1) Only subsystems can be added as variant choices at this level
      | 2) Blocks cannot be connected at this level as connectivity is
      | automatically determined at simulation, based on the active variant
  Bob : Subsystem  VariantControl=Bob
  Link : Subsystem  VariantControl=Link
  B : PMIOPort  Port=1  Side=Left
  F : PMIOPort  Port=2  Side=Right

== system Flexible_Beam_Compare/tictoc1 ==

== system Flexible_Beam_Compare/Flex Body State-Space/Deflection Joint ==
  Prismatic Joint1 : sm_lib/Joints/Prismatic Joint  SenseConstraintForce=off  SenseConstraintForceX=off  SenseConstraintForceY=off  SenseConstraintForceZ=off  SenseConstraintTorque=off  SenseConstraintTorqueX=off  SenseConstraintTorqueY=off  SenseConstraintTorqueZ=off  SenseTotalForce=off  SenseTotalForceX=off  SenseTotalForceY=off  SenseTotalForceZ=off  SenseTotalTorque=off  SenseTotalTorqueX=off  SenseTotalTorqueY=off  SenseTotalTorqueZ=off  CompositeWrenchDir=FollowerOnBase  CompositeWrenchFrame=BaseFrame  EquilibriumPosition=0  EquilibriumPositionUnits=m  SpringStiffness=0  SpringStiffnessUnits=N/m  DampingCoefficient=0  DampingCoefficientUnits=N/(m/s)  TorqueActuationMode=ComputedTorque  MotionActuationMode=InputMotion  SensePosition=off  SenseVelocity=off  SenseAcceleration=off  SenseTorqueForce=on  PositionTargetSpecify=off  PositionTargetPriority=High  PositionTargetValue=0  PositionTargetValueUnits=m  VelocityTargetSpecify=off  VelocityTargetPriority=High  VelocityTargetValue=0  VelocityTargetValueUnits=m/s
  Transform Beam6 : sm_lib/Frames and Transforms/Rigid Transform  TranslationMethod=None  TranslationLengthUnit=m  TranslationStandardAxis=+Z  TranslationStandardOffset=0  TranslationCartesianOffset=[0 0 0]  TranslationROffset=0  TranslationROffsetUnits=m  TranslationZOffset=0  TranslationZOffsetUnits=m  TranslationThetaOffset=0  TranslationThetaOffsetUnits=deg  RotationMethod=StandardAxis  RotationAngleUnits=deg  RotationStandardAxis=+X  RotationAngle=-90  RotationArbitraryAxis=[0 0 1]  FollAlignAxisA=+X  BaseAlignAxisA=+Y  FollAlignAxisB=+Y  BaseAlignAxisB=+Z  RotationSequenceAxes=FollowerAxes  RotationSequence=XYX  RotationSequenceAngles=[0 0 0]  RotationSequenceAnglesUnits=deg  RotationMatrix=[1 0 0; 0 1 0; 0 0 1]
  Transform Beam7 : sm_lib/Frames and Transforms/Rigid Transform  TranslationMethod=None  TranslationLengthUnit=m  TranslationStandardAxis=+Z  TranslationStandardOffset=0  TranslationCartesianOffset=[0 0 0]  TranslationROffset=0  TranslationROffsetUnits=m  TranslationZOffset=0  TranslationZOffsetUnits=m  TranslationThetaOffset=0  TranslationThetaOffsetUnits=deg  RotationMethod=StandardAxis  RotationAngleUnits=deg  RotationStandardAxis=+X  RotationAngle=90  RotationArbitraryAxis=[0 0 1]  FollAlignAxisA=+X  BaseAlignAxisA=+Y  FollAlignAxisB=+Y  BaseAlignAxisB=+Z  RotationSequenceAxes=FollowerAxes  RotationSequence=XYX  RotationSequenceAngles=[0 0 0]  RotationSequenceAnglesUnits=deg  RotationMatrix=[1 0 0; 0 1 0; 0 0 1]
  p : PMIOPort  Port=1  Side=Left
  f : PMIOPort  Port=2  Side=Right
  B : PMIOPort  Port=3  Side=Left
  F : PMIOPort  Port=4  Side=Right
  connections:
  Transform Beam6/RConn1 -- Prismatic Joint1/LConn1
  Transform Beam6/LConn1 -- B/RConn1
  Transform Beam7/RConn1 -- F/RConn1
  Prismatic Joint1/RConn1 -- Transform Beam7/LConn1
  Prismatic Joint1/LConn2 -- p/RConn1
  Prismatic Joint1/RConn2 -- f/RConn1

== system Flexible_Beam_Compare/Flex Body State-Space/Rigid Body ==
  Solid : sm_lib/Body Elements/Solid  InertiaType=CalculateFromGeometry  Mass=1  MassUnits=kg  CenterOfMass=[0 0 0]  CenterOfMassUnits=m  MomentsOfInertia=[1 1 1]  MomentsOfInertiaUnits=kg*m^2  ProductsOfInertia=[0 0 0]  ProductsOfInertiaUnits=kg*m^2  DensityBased=on  Density=density  DensityUnits=kg/(m^3)  DoExposeReferenceFrame=on  SerializedFrames=<Frames/>  GraphicType=FromGeometry  MarkerShape=Sphere  MarkerSize=10  MarkerSizeUnits=m  GraphicVisPropType=SimpleVisualProperties  GraphicDiffuseColor=[1.0 0.0 0.2]  GraphicSpecularColor=[0.5 0.5 0.5 1.0]  GraphicAmbientColor=[0.15 0.15 0.15 1.0]  GraphicEmissiveColor=[0.0 0.0 0.0 1.0]  GraphicShininess=75  GraphicOpacity=1.0  GeometryShape=GeneralExtrusion  RectangleSize=[1 1]  RectangleSizeUnits=m  BrickDimensions=[1 1 1]  BrickDimensionUnits=m  CylinderRadius=1  CylinderRadiusUnits=m  CylinderLength=1  CylinderLengthUnits=m  SphereRadius=1  SphereRadiusUnits=m  EllipsoidRadii=[1 1 1]  EllipsoidRadiiUnits=m  ExtrusionCrossSection=Extr_Data_Box(beam_width,beam_width-2*beam_wall,beam_width,beam_width-2*beam_wall)  ExtrusionCrossSectionUnits=m  ExtrusionLength=beam_length  ExtrusionLengthUnits=m  PolygonNumSides=3  PolygonOuterRadius=1  PolygonOuterRadiusUnits=m  ExtGeomFileType=STL  ExtGeomFileUnits=m  RevolutionCrossSection=[1 1; 1 -1; 2 -1; 2 1]  RevolutionCrossSectionUnits=m  RevolutionExtent=Full  RevolutionAngle=180  RevolutionAngleUnits=deg
  Transform BeamX1 : sm_lib/Frames and Transforms/Rigid Transform  TranslationMethod=StandardAxis  TranslationLengthUnit=m  TranslationStandardAxis=+Z  TranslationStandardOffset=0  TranslationCartesianOffset=[0 0 0]  TranslationROffset=0  TranslationROffsetUnits=m  TranslationZOffset=0  TranslationZOffsetUnits=m  TranslationThetaOffset=0  TranslationThetaOffsetUnits=deg  RotationMethod=StandardAxis  RotationAngleUnits=deg  RotationStandardAxis=+Y  RotationAngle=90  RotationArbitraryAxis=[0 0 1]  FollAlignAxisA=+X  BaseAlignAxisA=+Y  FollAlignAxisB=+Y  BaseAlignAxisB=+Z  RotationSequenceAxes=FollowerAxes  RotationSequence=XYX  RotationSequenceAngles=[0 0 0]  RotationSequenceAnglesUnits=deg  RotationMatrix=[1 0 0; 0 1 0; 0 0 1]
  Transform BeamX2 : sm_lib/Frames and Transforms/Rigid Transform  TranslationMethod=StandardAxis  TranslationLengthUnit=m  TranslationStandardAxis=+Z  TranslationStandardOffset=beam_length/2  TranslationCartesianOffset=[0 0 0]  TranslationROffset=0  TranslationROffsetUnits=m  TranslationZOffset=0  TranslationZOffsetUnits=m  TranslationThetaOffset=0  TranslationThetaOffsetUnits=deg  RotationMethod=None  RotationAngleUnits=deg  RotationStandardAxis=+Y  RotationAngle=90  RotationArbitraryAxis=[0 0 1]  FollAlignAxisA=+X  BaseAlignAxisA=+Y  FollAlignAxisB=+Y  BaseAlignAxisB=+Z  RotationSequenceAxes=FollowerAxes  RotationSequence=XYX  RotationSequenceAngles=[0 0 0]  RotationSequenceAnglesUnits=deg  RotationMatrix=[1 0 0; 0 1 0; 0 0 1]
  Transform BeamX3 : sm_lib/Frames and Transforms/Rigid Transform  TranslationMethod=StandardAxis  TranslationLengthUnit=m  TranslationStandardAxis=+Z  TranslationStandardOffset=beam_length/2  TranslationCartesianOffset=[0 0 0]  TranslationROffset=0  TranslationROffsetUnits=m  TranslationZOffset=0  TranslationZOffsetUnits=m  TranslationThetaOffset=0  TranslationThetaOffsetUnits=deg  RotationMethod=None  RotationAngleUnits=deg  RotationStandardAxis=+Y  RotationAngle=90  RotationArbitraryAxis=[0 0 1]  FollAlignAxisA=+X  BaseAlignAxisA=+Y  FollAlignAxisB=+Y  BaseAlignAxisB=+Z  RotationSequenceAxes=FollowerAxes  RotationSequence=XYX  RotationSequenceAngles=[0 0 0]  RotationSequenceAnglesUnits=deg  RotationMatrix=[1 0 0; 0 1 0; 0 0 1]
  B : PMIOPort  Port=1  Side=Left
  F : PMIOPort  Port=2  Side=Right
  connections:
  Transform BeamX1/RConn1 -- Transform BeamX2/LConn1
  F/RConn1 -- Transform BeamX3/RConn1
  Transform BeamX2/RConn1 -- Solid/RConn1 -- Transform BeamX3/LConn1
  Transform BeamX1/LConn1 -- B/RConn1

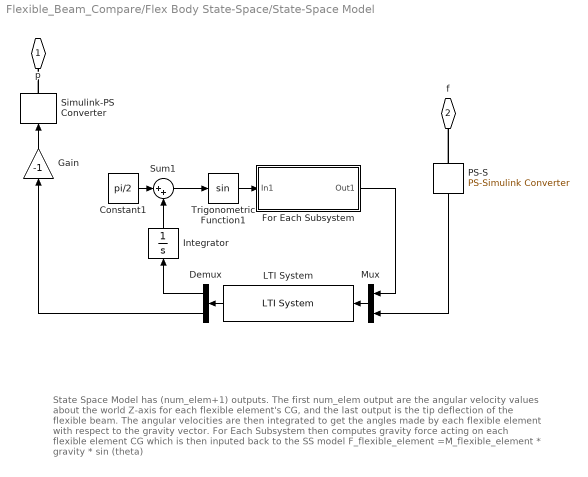
== system Flexible_Beam_Compare/Flex Body State-Space/State-Space Model ==
  note: State Space Model has (num_elem+1) outputs.
      | The first num_elem output are the angular velocity values about the world Z-axis for each flexible
      | element's CG, and the last output is the tip deflection of the flexible beam.
      | The angular velocities are then integrated to get the angles made by each flexible element with
      | respect to the gravity vector.
      | For Each Subsystem then computes gravity force acting on each flexible element CG which is
      | then inputed back to the SS model
      |
      | F_flexible_element =M_flexible_element * gravity * sin (theta)
  Constant1 : Constant  Value=pi/2
  Demux : Demux  Outputs=[num_elem 1]
  For Each Subsystem : Subsystem  TreatAsAtomicUnit=on
  Gain : Gain  Gain=-1
  Integrator : Integrator
  LTI System : cstblocks/LTI System  sys=linsys_beam_fixfree  IC=[]
  Mux : Mux  Inputs=2
  PS-S : nesl_utility/PS-Simulink Converter  PhysicalDomain=network_engine_domain  SubClassName=ps_output  LeftPortType=input  RightPortType=output  PseudoPeriodic=off  Frequencies=[]  Unit=1  AffineConversion=off
  Simulink-PS Converter : nesl_utility/Simulink-PS Converter  PhysicalDomain=network_engine_domain  SubClassName=ps_input  LeftPortType=input  RightPortType=output  PseudoPeriodic=off  Frequencies=[]  NoiseDistribution=none  NoiseParameters=[]  Unit=1  AffineConversion=off  InputFiltering=on  SimscapeFilterOrder=2  InputFilterTimeConstant=1e-3  UdotUserProvided=1
  Sum1 : Sum  Inputs=|++
  Trigonometric Function1 : Trigonometry
  p : PMIOPort  Port=1  Side=Right
  f : PMIOPort  Port=2  Side=Left
  wires:
  Gain/1 -> Simulink-PS Converter/1
  Mux/1 -> LTI System/1
  PS-S/1 -> Mux/2
  Demux/2 -> Gain/1
  For Each Subsystem/1(Out1) -> Mux/1
  LTI System/1 -> Demux/1
  Sum1/1 -> Trigonometric Function1/1
  Trigonometric Function1/1 -> For Each Subsystem/1(In1)
  Constant1/1 -> Sum1/1
  Integrator/1 -> Sum1/2
  Demux/1 -> Integrator/1
  connections:
  PS-S/LConn1 -- f/RConn1
  Simulink-PS Converter/RConn1 -- p/RConn1
